simulink model "distillationProcess"  (R2023b)
settings: Solver=VariableStepAuto  StartTime=0.0  StopTime=1800  RelTol=1e-6
libraries: cstblocks x4
settings Model: Creator=alfredo  LastModifiedBy=roberto_ambrosino
settings SolverCC: AlgebraicLoopSolver=TrustRegion
settings DebuggingCC: UnconnectedInputMsg=warning  UnconnectedOutputMsg=warning  UnconnectedLineMsg=warning
settings ModelReferenceCC: EnableRefExpFcnMdlSchedulingChecks=on

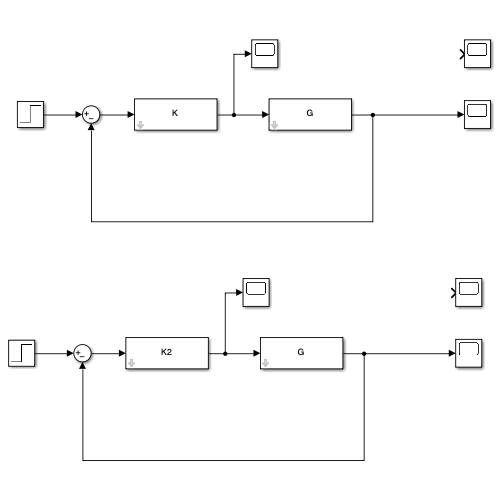
[thumbnail: Simulink's stored preview of the top-level diagram]
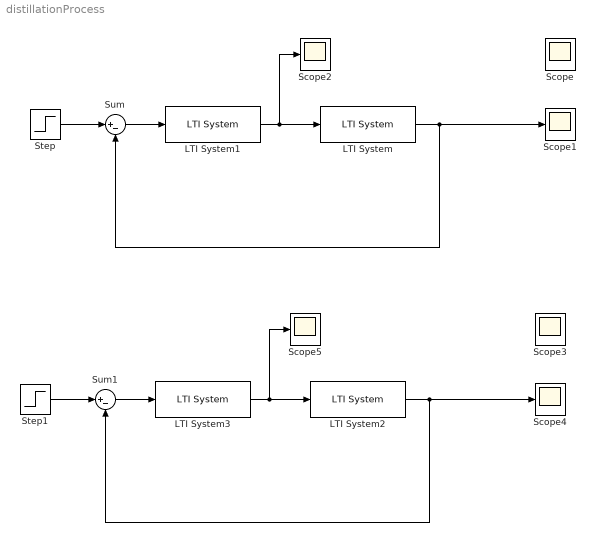
== system distillationProcess ==
  LTI System : cstblocks/LTI System  sys=G  IC=[]  PadeOrder=0
  LTI System1 : cstblocks/LTI System  sys=K  IC=[]  PadeOrder=0
  LTI System2 : cstblocks/LTI System  sys=G  IC=[]  PadeOrder=0
  LTI System3 : cstblocks/LTI System  sys=K2  IC=[]  PadeOrder=0
  Scope{,1..5} (6 alike) : Scope
  Step : Step  Time=0  Before=[0;0]  After=[1;0.6]  SampleTime=0
  Step1 : Step  Time=0  Before=[0;0]  After=[1;0.6]  SampleTime=0
  Sum : Sum  Inputs=|+-
  Sum1 : Sum  Inputs=|+-
  wires:
  LTI System1/1 -> Scope2/1, LTI System/1
  Step/1 -> Sum/1
  Sum/1 -> LTI System1/1
  LTI System/1 -> Scope1/1, Sum/2
  Sum1/1 -> LTI System3/1
  LTI System2/1 -> Scope4/1, Sum1/2
  Step1/1 -> Sum1/1
  LTI System3/1 -> Scope5/1, LTI System2/1
